simulink model "helicopter_MPC_21b"  (R2021b)
settings: Solver=FixedStepAuto  StartTime=0.0  StopTime=60  FixedStep=0.001  RelTol=1e-3
InitFcn:
  | hwinit
StopFcn:
  | helicoptertest_plot
values from neighbouring files (symbols this model uses):
  Ac_neg = Ac    [hwinit.m]
  Ac_pos = Ac    [hwinit.m]
  adingain = [pitchgain 1 yawgain 1]    [hwinit.m]
  adinoffs = [pitchoffs 0 yawoffs 0]    [hwinit.m]
  angle_ref = neg.mean.pitch(idx)    [hwinit.m]
  angVel_ref = neg.mean.angular_velocity(idx)    [hwinit.m]
  bc_neg = bc    [hwinit.m]
  bc_pos = bc    [hwinit.m]
  F_neg = F    [hwinit.m]
  F_pos = F    [hwinit.m]
  h = 0.001    [hwinit.m]
  input_ref = -0.5    [hwinit.m]
  Linv_neg = Linv    [hwinit.m]
  Linv_pos = Linv    [hwinit.m]
undefined symbols (not defined in the file or in its folder): helicopterSysID_neg, helicopterSysID_pos, HeliMexHandle, L_neg, L_pos
libraries: dspfdesign x1
settings Model: Creator=fkzhang  LastModifiedBy=morhun
settings SolverCC: AlgebraicLoopSolver=TrustRegion
settings DataIOCC: LimitDataPoints=on  SaveFormat=Array  ReturnWorkspaceOutputs=off
settings OptimizationCC: BlockReduction=off  BooleanDataType=off  LifeSpan=inf
settings DebuggingCC: SaveWithParameterizedLinksMsg=none  UnderspecifiedInitializationDetection=Classic  MergeDetectMultiDrivingBlocksExec=none  SignalResolutionControl=TryResolveAllWithWarning  AllowSymbolicDim=off  SFUnexpectedBacktrackingDiag=warning  SFNoUnconditionalDefaultTransitionDiag=warning  SFExecutionAtInitializationDiag=none  ArithmeticOperatorsInVariantConditions=warning
settings HardwareCC: ProdBitPerPointer=32  ProdBitPerSizeT=32  ProdBitPerPtrDiffT=32  ProdLargestAtomicFloat=None  ProdIntDivRoundTo=Undefined  ProdEndianess=Unspecified  ProdWordSize=32  ProdHWDeviceType=32-bit Generic  TargetBitPerPointer=64  TargetBitPerSizeT=64  TargetBitPerPtrDiffT=64  TargetLongLongMode=on  TargetIntDivRoundTo=Zero  TargetEndianess=LittleEndian  TargetWordSize=64  TargetHWDeviceType=MATLAB Host  ProdEqTarget=off
settings ModelReferenceCC: PropagateSignalLabelsOutOfModel=off
settings SFSimCC: SimUseLocalCustomCode=off  CustomCodeUndefinedFunction=UseInterfaceOnly
settings RTWCC: RTWUseLocalCustomCode=off
settings CodeAppCC: StateflowObjectComments=on
settings GRTTargetCC: TargetLangStandard=C89/C90 (ANSI)
settings ConfigComp: CovMetricSettings=dw  CovSaveCumulativeToWorkspaceVar=on  CovSaveSingleToWorkspaceVar=on  CovExternalEMLEnable=off  CovSFcnEnable=off

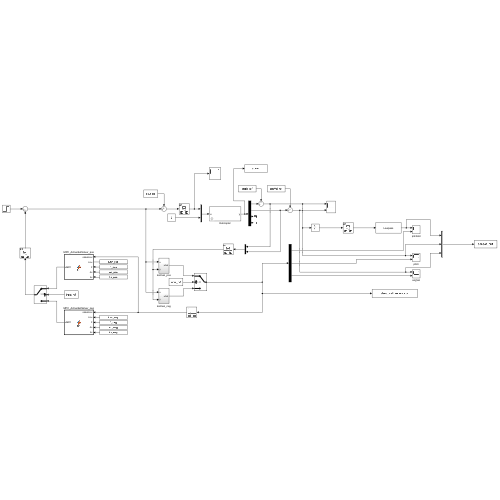
[thumbnail: Simulink's stored preview of the top-level diagram]
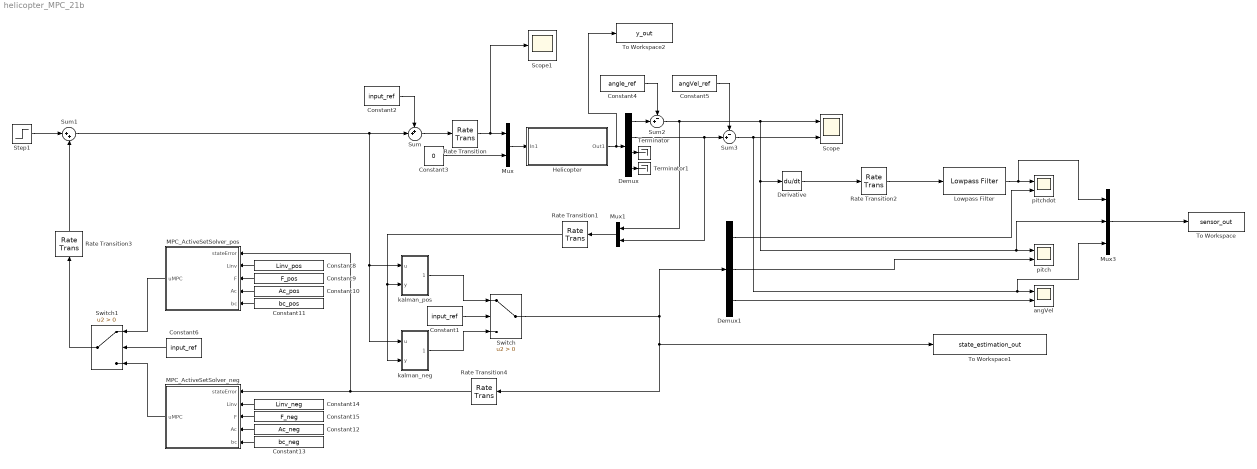
== system helicopter_MPC_21b ==
  Constant1 : Constant  Value=input_ref
  Constant10 : Constant  Value=Ac_pos  VectorParams1D=off
  Constant11 : Constant  Value=bc_pos  VectorParams1D=off
  Constant12 : Constant  Value=Ac_neg  VectorParams1D=off
  Constant13 : Constant  Value=bc_neg  VectorParams1D=off
  Constant14 : Constant  Value=Linv_neg  VectorParams1D=off
  Constant15 : Constant  Value=F_neg  VectorParams1D=off
  Constant2 : Constant  Value=input_ref
  Constant3 : Constant  Value=0
  Constant4 : Constant  Value=angle_ref  SampleTime=h
  Constant5 : Constant  Value=angVel_ref  SampleTime=h
  Constant6 : Constant  Value=input_ref
  Constant8 : Constant  Value=Linv_pos  VectorParams1D=off
  Constant9 : Constant  Value=F_pos  VectorParams1D=off
  Demux : Demux
  Demux1 : Demux  Outputs=3
  Derivative : Derivative
  Helicopter : Subsystem  mask{Ts=h}
      mask prompts: Ts "sampletime"
      mask init:
      | sf_heli_init
      mask Display:
      | port_label('input',1,'u');
      | port_label('output',1,'y');
  Lowpass Filter : dspfdesign/Lowpass Filter  FilterType=FIR  DesignForMinimumOrder=on  FilterOrder=50  PassbandFrequency=1  StopbandFrequency=10  PassbandRipple=0.1  StopbandAttenuation=80  InheritSampleRate=off  SampleRate=1000  SimulateUsing=Interpreted execution  roundingMode=Floor  coeffsDataTypeStr=fixdt(1,16)
  MPC_ActiveSetSolver_neg : MATLAB Function  TreatAsAtomicUnit=on
  MPC_ActiveSetSolver_pos : MATLAB Function  TreatAsAtomicUnit=on
  Mux : Mux  Inputs=2
  Mux1 : Mux  Inputs=2
  Mux3 : Mux  Inputs=3
  Rate Transition : RateTransition  OutPortSampleTime=h
  Rate Transition1 : RateTransition
  Rate Transition2 : RateTransition  OutPortSampleTime=h
  Rate Transition3 : RateTransition
  Rate Transition4 : RateTransition  OutPortSampleTime=h
  Scope : Scope  NumInputPorts=2
  Scope1 : Scope
  Step1 : Step  Time=0  After=0  SampleTime=0
  Sum : Sum  Inputs=++|
  Sum1 : Sum  Inputs=|++
  Sum2 : Sum  Inputs=-+|
  Sum3 : Sum  Inputs=-+|
  Switch : Switch  Criteria=u2 > Threshold
  Switch1 : Switch  Criteria=u2 > Threshold
  Terminator : Terminator
  Terminator1 : Terminator
  To Workspace : ToWorkspace  VariableName=sensor_out  SaveFormat=Timeseries  SampleTime=-1
  To Workspace1 : ToWorkspace  VariableName=state_estimation_out  SaveFormat=Timeseries  SampleTime=-1
  To Workspace2 : ToWorkspace  VariableName=y_out  SaveFormat=Timeseries  SampleTime=-1
  angVel : Scope  NumInputPorts=2
  kalman_neg : Subsystem
  kalman_pos : Subsystem
  pitch : Scope  NumInputPorts=2
  pitchdot : Scope  NumInputPorts=2
  wires:
  Mux/1 -> Helicopter/1(In1)
  Constant3/1 -> Mux/2
  Sum1/1 -> kalman_neg/1(u), kalman_pos/1(u), Sum/2
  Switch/1 -> To Workspace1/1, Rate Transition4/1, Demux1/1
  Constant2/1 -> Sum/1
  Demux/3 -> Terminator/1
  Demux/4 -> Terminator1/1
  Demux/1 -> Sum2/2
  Demux/2 -> Mux1/2, Sum3/2
  Constant4/1 -> Sum2/1
  Constant5/1 -> Sum3/1
  Constant1/1 -> Switch/2
  kalman_pos/1(xhat) -> Switch/1
  kalman_neg/1(xhat) -> Switch/3
  Rate Transition2/1 -> Lowpass Filter/1
  Derivative/1 -> Rate Transition2/1
  Mux1/1 -> Rate Transition1/1
  Rate Transition1/1 -> kalman_neg/2(y), kalman_pos/2(y)
  Demux1/1 -> pitchdot/2
  Demux1/2 -> pitch/2
  Demux1/3 -> angVel/2
  Sum/1 -> Rate Transition/1
  Constant6/1 -> Switch1/2
  MPC_ActiveSetSolver_pos/1(uMPC) -> Switch1/1
  MPC_ActiveSetSolver_neg/1(uMPC) -> Switch1/3
  Step1/1 -> Sum1/1
  Constant8/1 -> MPC_ActiveSetSolver_pos/2(Linv)
  Constant9/1 -> MPC_ActiveSetSolver_pos/3(F)
  Constant10/1 -> MPC_ActiveSetSolver_pos/4(Ac)
  Constant11/1 -> MPC_ActiveSetSolver_pos/5(bc)
  Constant14/1 -> MPC_ActiveSetSolver_neg/2(Linv)
  Constant15/1 -> MPC_ActiveSetSolver_neg/3(F)
  Constant12/1 -> MPC_ActiveSetSolver_neg/4(Ac)
  Constant13/1 -> MPC_ActiveSetSolver_neg/5(bc)
  Rate Transition/1 -> Scope1/1, Mux/1
  Sum2/1 -> Mux1/1, pitch/1, Mux3/2, Derivative/1, Scope/1
  Sum3/1 -> Mux3/3, angVel/1, Scope/2
  Mux3/1 -> To Workspace/1
  Lowpass Filter/1 -> Mux3/1, pitchdot/1
  Helicopter/1(Out1) -> To Workspace2/1, Demux/1
  Switch1/1 -> Rate Transition3/1
  Rate Transition3/1 -> Sum1/2
  Rate Transition4/1 -> MPC_ActiveSetSolver_pos/1(stateError), MPC_ActiveSetSolver_neg/1(stateError)

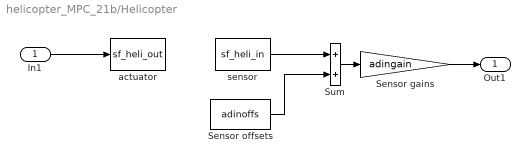
== system helicopter_MPC_21b/Helicopter ==
  In1 : Inport
  Sensor gains : Gain  Gain=adingain
  Sensor offsets : Constant  Value=adinoffs
  Sum : Sum
  actuator : M-S-Function  FunctionName=sf_heli_out  Parameters=HeliMexHandle,Ts
  sensor : M-S-Function  FunctionName=sf_heli_in  Parameters=HeliMexHandle
  Out1 : Outport
  wires:
  sensor/1 -> Sum/1
  In1/1 -> actuator/1
  Sensor offsets/1 -> Sum/2
  Sum/1 -> Sensor gains/1
  Sensor gains/1 -> Out1/1

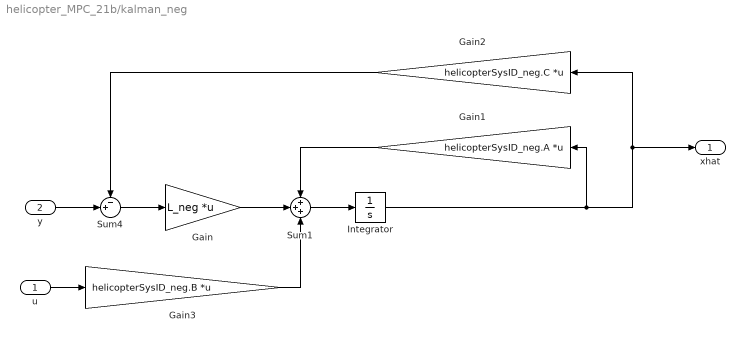
== system helicopter_MPC_21b/kalman_neg ==
  u : Inport
  y : Inport  Port=2
  Gain : Gain  Gain=L_neg  Multiplication=Matrix(K*u)
  Gain1 : Gain  Gain=helicopterSysID_neg.A  Multiplication=Matrix(K*u)
  Gain2 : Gain  Gain=helicopterSysID_neg.C  Multiplication=Matrix(K*u)
  Gain3 : Gain  Gain=helicopterSysID_neg.B  Multiplication=Matrix(K*u)
  Integrator : Integrator  InitialCondition=[0 ; -angle_ref ; -angVel_ref]
  Sum1 : Sum  Inputs=+++
  Sum4 : Sum  Inputs=-+|
  xhat : Outport
  wires:
  Integrator/1 -> Gain1/1, xhat/1, Gain2/1
  y/1 -> Sum4/2
  Sum4/1 -> Gain/1
  u/1 -> Gain3/1
  Gain3/1 -> Sum1/3
  Gain/1 -> Sum1/2
  Sum1/1 -> Integrator/1
  Gain1/1 -> Sum1/1
  Gain2/1 -> Sum4/1

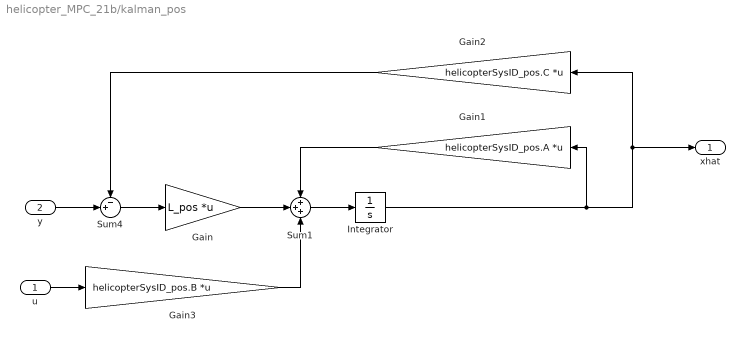
== system helicopter_MPC_21b/kalman_pos ==
  u : Inport
  y : Inport  Port=2
  Gain : Gain  Gain=L_pos  Multiplication=Matrix(K*u)
  Gain1 : Gain  Gain=helicopterSysID_pos.A  Multiplication=Matrix(K*u)
  Gain2 : Gain  Gain=helicopterSysID_pos.C  Multiplication=Matrix(K*u)
  Gain3 : Gain  Gain=helicopterSysID_pos.B  Multiplication=Matrix(K*u)
  Integrator : Integrator  InitialCondition=[0 ; -angle_ref ; -angVel_ref]
  Sum1 : Sum  Inputs=+++
  Sum4 : Sum  Inputs=-+|
  xhat : Outport
  wires:
  Integrator/1 -> Gain1/1, xhat/1, Gain2/1
  y/1 -> Sum4/2
  Sum4/1 -> Gain/1
  u/1 -> Gain3/1
  Gain3/1 -> Sum1/3
  Gain/1 -> Sum1/2
  Sum1/1 -> Integrator/1
  Gain1/1 -> Sum1/1
  Gain2/1 -> Sum4/1

== matlab function helicopter_MPC_21b/MPC_ActiveSetSolver_pos ==
  data: stateError input; uMPC output; Linv input; F input; Ac input; bc input
function uMPC = fcn(stateError,Linv,F,Ac,bc)
    % coder.extrinsic('mpcActiveSetSolver');
    stateErrorV = zeros(3,1);
    stateErrorV(1) = stateError(1);
    stateErrorV(2) = stateError(2);
    stateErrorV(3) = stateError(3);

    iA = false(size(bc));
    opt = mpcActiveSetOptions;
    opt.UseHessianAsInput=false;
    opt.IntegrityChecks=false;

    MPC = mpcActiveSetSolver(Linv,F*stateErrorV,Ac,bc,zeros(0,width(Ac)),zeros(0,1),iA,opt);
    uMPC = MPC(1,1);

== matlab function helicopter_MPC_21b/MPC_ActiveSetSolver_neg ==
  data: stateError input; uMPC output; Linv input; F input; Ac input; bc input
function uMPC = fcn(stateError,Linv,F,Ac,bc)
    % coder.extrinsic('mpcActiveSetSolver');
    stateErrorV = zeros(3,1);
    stateErrorV(1) = stateError(1);
    stateErrorV(2) = stateError(2);
    stateErrorV(3) = stateError(3);

    iA = false(size(bc));
    opt = mpcActiveSetOptions;
    opt.UseHessianAsInput=false;
    opt.IntegrityChecks=false;

    MPC = mpcActiveSetSolver(Linv,F*stateErrorV,Ac,bc,zeros(0,width(Ac)),zeros(0,1),iA,opt);
    uMPC = MPC(1,1);
